simulink model "SF5_5_1_jc0750"  (R2016b)
settings: Solver=VariableStepAuto  StartTime=0.0  StopTime=10.0  RelTol=1e-3  EnableMultiTasking=on
settings Model: Creator=amyyang  LastModifiedBy=amyyang
settings DataIOCC: LimitDataPoints=on
settings OptimizationCC: LifeSpan=inf
settings DebuggingCC: AllowSymbolicDim=off  SFUnexpectedBacktrackingDiag=warning  SFNoUnconditionalDefaultTransitionDiag=warning  SFExecutionAtInitializationDiag=none
settings ModelReferenceCC: PropagateSignalLabelsOutOfModel=off
settings GRTTargetCC: TargetLangStandard=C89/C90 (ANSI)
settings ConfigComp: CovMetricSettings=dw  CovHtmlReporting=on  CovSaveCumulativeToWorkspaceVar=on  CovSaveSingleToWorkspaceVar=on  CovExternalEMLEnable=off

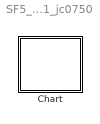
== system SF5_5_1_jc0750 ==
  Chart : Stateflow chart  TreatAsAtomicUnit=on

== stateflow chart SF5_5_1_jc0750/Chart ==
  state Correct
    entry:
    a = 0;
    b = 0;
    during:
    a = a + in1;
    b = a * 2;
  state S10
    during:
    a = a + in1;
    b = a * 2;
  note: 要么垂直，要么水平
  state Correct1
    entry:
    a = 0;
    b = 0;
    during:
    a = a + in1;
    b = a * 2;
  state InCorrect2
    entry:
    a = 0;
    b = 0;
    during:
    a = a + in1;
    b = a * 2;
  state S11
    during:
    a = a + in1;
    b = a * 2;
  state S12
    during:
    a = a + in1;
    b = a * 2;
  (default) -> Correct [order 1]
  Correct -> S10 : [after(10,sec)]
      | {
      | c = b;
      | }
  S10 -> Correct : [after(10,sec)]
      | {
      | c = b;
      | }
  (default) -> Correct1 [order 2]
  (default) -> InCorrect2 [order 3]
  S12 -> InCorrect2 : [after(10,sec)]
      | {
      |  c = b;
      | }
  InCorrect2 -> S12 : [after(10,sec)]
      | {
      |  c = b;
      | }
  Correct1 -> S11 : [after(10,sec)]
      | {
      |  c = b;
      | }
  S11 -> Correct1 : [after(10,sec)]
      | {
      |  c = b;
      | }
